simulink model "rate_limiter_integrator_compensator"  (R2015b)
settings: Solver=VariableStepAuto  StartTime=0.0  StopTime=100.0  FixedStep=1e-3  MaxStep=1e-6  MinStep=1e-6  RelTol=1e-6
settings Model: Creator=dell  LastModifiedBy=dell

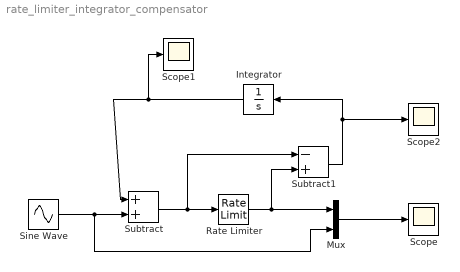
== system rate_limiter_integrator_compensator ==
  Integrator : Integrator
  Mux : Mux  Inputs=2
  Rate Limiter : RateLimiter  SampleTimeMode=inherited
  Scope : Scope
  Scope1 : Scope
  Scope2 : Scope
  Sine Wave : Sin  Amplitude=5  SampleTime=0
  Subtract : Sum
  Subtract1 : Sum  Inputs=-+
  wires:
  Subtract/1 -> Subtract1/1, Rate Limiter/1
  Rate Limiter/1 -> Mux/1, Subtract1/2
  Subtract1/1 -> Scope2/1, Integrator/1
  Integrator/1 -> Scope1/1, Subtract/1
  Sine Wave/1 -> Mux/2, Subtract/2
  Mux/1 -> Scope/1
